simulink model "modelExperiment_QuanserAero_Hardware_AdaptiveV5"  (R2021a)
settings: Solver=ode1  StartTime=0.0  StopTime=T  FixedStep=DAQ_time  RelTol=1e-3  EnableMultiTasking=on
PreLoadFcn:
  | quanser_aero_lqr
values from neighbouring files (symbols this model uses):
  A_cmd = [Ap_cmd, Ay_cmd]    [runExperiment_QuanserAero_Hardware_AdaptiveV4_1DOF_pitch.m]    (also in runExperiment_QuanserAero_Hardware_AdaptiveV4_1DOF_yaw.m; runSim_QuanserAero_AdaptiveV3.m; run_QuanserAero_AdaptiveV3_SN.m)
  a_cmd_coeff = [ap_cmd_coeff,ay_cmd_coeff]    [runExperiment_QuanserAero_Hardware_AdaptiveV4_1DOF_pitch.m]    (also in runExperiment_QuanserAero_Hardware_AdaptiveV4_1DOF_yaw.m; runSim_QuanserAero_AdaptiveV3.m; run_QuanserAero_AdaptiveV3_SN.m)
  cmd_select = [1,0]    [runExperiment_QuanserAero_Hardware_AdaptiveV4_1DOF_pitch.m]    (also in runExperiment_QuanserAero_Hardware_AdaptiveV4_1DOF_yaw.m = [1,1]; runSim_QuanserAero_AdaptiveV3.m = [0,2]; run_QuanserAero_AdaptiveV3_SN.m = [0,2])
  control_gains = [lambda_p lambda_y ... (first row only)    [runExperiment_QuanserAero_Hardware_AdaptiveV4_1DOF_pitch.m]    (also in runExperiment_QuanserAero_Hardware_AdaptiveV4_1DOF_yaw.m; runSim_QuanserAero_AdaptiveV3.m; run_QuanserAero_AdaptiveV3_SN.m)
  gamma_p = [gamma0_p;gamma1_p;gamma2_p;gamma3_p;gamma4_p]    [runExperiment_QuanserAero_Hardware_AdaptiveV4_1DOF_pitch.m]    (also in runExperiment_QuanserAero_Hardware_AdaptiveV4_1DOF_yaw.m; runSim_QuanserAero_AdaptiveV3.m; run_QuanserAero_AdaptiveV3_SN.m)
  gamma_y = [gamma0_y;gamma1_y;gamma2_y;gamma3_y]    [runExperiment_QuanserAero_Hardware_AdaptiveV4_1DOF_pitch.m]    (also in runExperiment_QuanserAero_Hardware_AdaptiveV4_1DOF_yaw.m; runSim_QuanserAero_AdaptiveV3.m; run_QuanserAero_AdaptiveV3_SN.m)
  harmonic_cutoff_p = Tp_cmd*harmonic_cycles    (= 20)    [runExperiment_QuanserAero_Hardware_AdaptiveV4_1DOF_pitch.m]    (also in runExperiment_QuanserAero_Hardware_AdaptiveV4_1DOF_yaw.m; runSim_QuanserAero_AdaptiveV3.m; run_QuanserAero_AdaptiveV3_SN.m)
  harmonic_cutoff_y = Ty_cmd*harmonic_cycles    (= 20)    [runExperiment_QuanserAero_Hardware_AdaptiveV4_1DOF_pitch.m]    (also in runExperiment_QuanserAero_Hardware_AdaptiveV4_1DOF_yaw.m; runSim_QuanserAero_AdaptiveV3.m; run_QuanserAero_AdaptiveV3_SN.m = 40)
  paramsGuess_haaaa = [hp_hat hy_hat ... (first row only)    [runExperiment_QuanserAero_Hardware_AdaptiveV4_1DOF_pitch.m]    (also in runExperiment_QuanserAero_Hardware_AdaptiveV4_1DOF_yaw.m; runSim_QuanserAero_AdaptiveV3.m; run_QuanserAero_AdaptiveV3_SN.m)
  T_cmd = [Tp_cmd, Ty_cmd]    [runExperiment_QuanserAero_Hardware_AdaptiveV4_1DOF_pitch.m]    (also in runExperiment_QuanserAero_Hardware_AdaptiveV4_1DOF_yaw.m; runSim_QuanserAero_AdaptiveV3.m; run_QuanserAero_AdaptiveV3_SN.m)
  time_offset = 2    [runExperiment_QuanserAero_Hardware_AdaptiveV4_1DOF_pitch.m]    (also in runExperiment_QuanserAero_Hardware_AdaptiveV4_1DOF_yaw.m)
undefined symbols (not defined in the file or in its folder): HIL, qc_get_step_size
libraries: quarc_library x7
settings Model: SimulationMode=external  ExtModeTrigDuration=20000  Creator=MLevis  LastModifiedBy=Student
settings SolverCC: AlgebraicLoopSolver=TrustRegion  PositivePriorityOrder=on
settings DataIOCC: LimitDataPoints=on  SaveFormat=Array  ReturnWorkspaceOutputs=off
settings DebuggingCC: SolverPrmCheckMsg=warning  SFUnexpectedBacktrackingDiag=warning  SFNoUnconditionalDefaultTransitionDiag=warning  SFExecutionAtInitializationDiag=none  SFMachineParentedDataDiag=warning  ArithmeticOperatorsInVariantConditions=warning
settings ModelReferenceCC: PropagateSignalLabelsOutOfModel=off
settings SFSimCC: SimUseLocalCustomCode=off  CustomCodeUndefinedFunction=UseInterfaceOnly
settings RTWCC: Description=QUARC Win64 Target Using Toolchain  SystemTargetFile=quarc_win64.tlc  TemplateMakefile=quarc_default_tmf  RTWUseLocalCustomCode=off  Toolchain=QUARC win64 | nmake (64-bit Windows)  BuildConfiguration=Faster Runs
settings CodeAppCC: StateflowObjectComments=on
settings STFCustomTargetCC: ConcurrentExecutionCompliant=on  SystemTargetFile=quarc_win64.tlc
settings GRTTargetCC: TargetLangStandard=C89/C90 (ANSI)  ParMdlRefBuildCompliant=off  CompOptLevelCompliant=off  CombineOutputUpdateFcns=off  MatFileLogging=off  CPPClassGenCompliant=off  GRTInterface=on  ExtMode=on  ExtModeMexFile=quarc_comm
settings ConfigComp: CovMetricSettings=dw  CovSaveCumulativeToWorkspaceVar=on  CovSaveSingleToWorkspaceVar=on  CovExternalEMLEnable=off  CovSFcnEnable=off

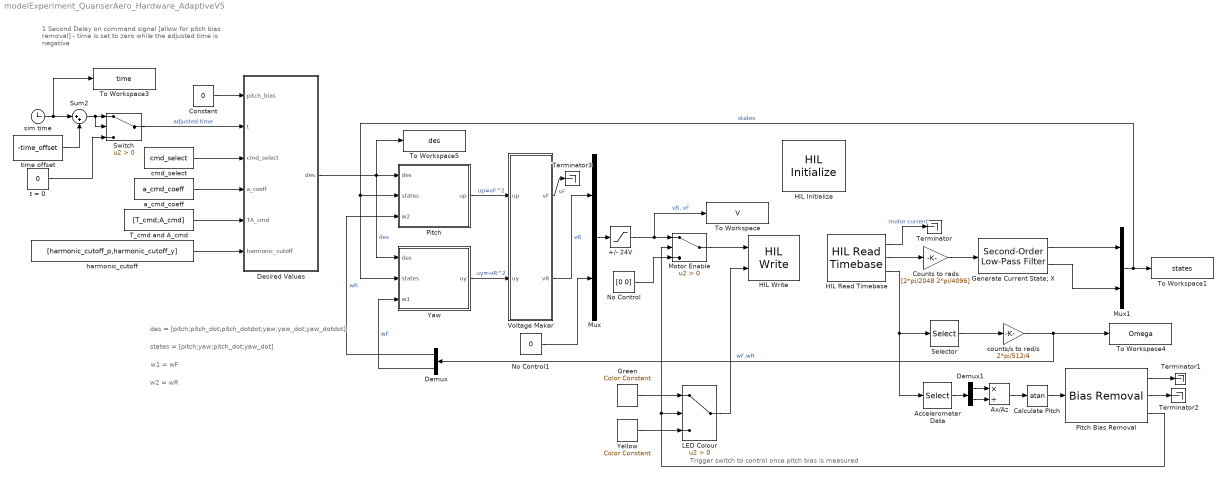
== system modelExperiment_QuanserAero_Hardware_AdaptiveV5 ==
  note: des = [pitch;pitch_dot;pitch_dotdot;yaw;yaw_dot;yaw_dotdot]
  note: w2 = wR
  note: w1 = wF
  note: 1 Second Delay on command signal
      | [allow for pitch bias removal]
      | - time is set to zero while the adjusted time is negative
  note: Trigger switch to control once pitch bias is measured
  note: states = [pitch;yaw;pitch_dot;yaw_dot]
  +/- 24V : Saturate  UpperLimit=24  LowerLimit=-24
  Accelerometer Data : Selector  InputPortWidth=4  IndexOptions=Index vector (dialog)  Indices=[1 2]  OutputSizes=1
  Ax/Az : Product  Inputs=*/
  Calculate Pitch : Trigonometry  Operator=atan
  Constant : Constant  Value=0
  Counts to rads : Gain  Gain=[2*pi/2048 2*pi/4096]
  Demux : Demux  Outputs=2
  Demux1 : Demux  Outputs=2
  Desired Values : MATLAB Function  TreatAsAtomicUnit=on
  Generate Current State; X : quarc_library/Continuous/Second-Order Low-Pass Filter  params_source=Internal (dialog parameters)  input_width=50  input_zeta=0.8  input_init=0
  Green : quarc_library/Sources/Signals/Color Constant  color=[0 1 0]
      settings: SourceProductName=QUARC Targets
  HIL Initialize : quarc_library/Data Acquisition/Generic/Configuration/HIL Initialize  Priority=-99  object_name=HIL-1  board_type=quanser_aero_usb  board_number=0  board_options=""  exclusive=off  active=off  hardware_clocks=[0]  clock_modes=[]  initial_clock_frequencies=[]  set_clock_params_at_start=off  set_clock_params_at_switch_in=off  set_clock_frequencies_at_start=off  set_clock_frequencies_at_switch_in=off  analog_input_channels=[0:1]  analog_input_configurations=[]  analog_input_maximums=3  analog_input_minimums=-3  set_analog_input_params_at_start=off  set_analog_input_params_at_switch_in=off  analog_output_channels=[0:1]  analog_output_maximums=24  analog_output_minimums=-24  initial_analog_outputs=[0]  final_analog_outputs=[0]  watchdog_analog_outputs=[0]  set_analog_output_params_at_start=off  set_analog_output_params_at_switch_in=off  set_analog_outputs_at_start=on  set_analog_outputs_at_switch_in=off  set_analog_outputs_at_terminate=on  set_analog_outputs_at_switch_out=off  set_analog_outputs_on_watchdog=on  digital_input_channels=[]  digital_output_channels=[0:1]  digital_output_configuration=[]  initial_digital_outputs=[1]  final_digital_outputs=[0]  watchdog_digital_outputs=[0]  set_digital_output_params_at_start=off  set_digital_output_params_at_switch_in=off  set_digital_outputs_at_start=on  set_digital_outputs_at_switch_in=off  set_digital_outputs_at_terminate=on  set_digital_outputs_at_switch_out=off  set_digital_outputs_on_watchdog=on  encoder_channels=[0:3]  quadrature=[4]  encoder_filter_frequency=[]  initial_encoder_counts=[0]  set_encoder_params_at_start=off  set_encoder_params_at_switch_in=off  set_encoder_counts_at_start=on  set_encoder_counts_at_switch_in=off  pwm_channels=[]  pwm_modes=[]  pwm_frequency=[]  pwm_configuration=[]  pwm_alignment=[]  pwm_polarity=[]  pwm_leading_deadband=[]  pwm_trailing_deadband=[]  initial_pwm_outputs=[]  final_pwm_outputs=[]  watchdog_pwm_outputs=[]  set_pwm_params_at_start=off  set_pwm_params_at_switch_in=off  set_pwm_outputs_at_start=off  set_pwm_outputs_at_switch_in=off  set_pwm_outputs_at_terminate=off  set_pwm_outputs_at_switch_out=off  set_pwm_outputs_on_watchdog=off  other_output_channels=[11000:11002]  initial_other_outputs=[0 1 0]  final_other_outputs=[1 0 0]  watchdog_other_outputs=[0 0 1]  set_other_outputs_at_start=on  set_other_outputs_at_switch_in=off  set_other_outputs_at_terminate=on  set_other_outputs_at_switch_out=off  set_other_outputs_on_watchdog=on
  HIL Read Timebase : quarc_library/Data Acquisition/Generic/Timebases/HIL Read Timebase  object_name=HIL-1  clock=0  analog_channels=[0:1]  encoder_channels=[2:3]  digital_channels=[]  other_channels=[4000 4002 14000 14001]  active=on  vector_output=on  data_type_mode=Inherit via back propagation  encoder_data_type=double  digital_data_type=boolean  overflow_mode=Error on overflow  samples_in_buffer=max(ceil(1/qc_get_step_size), 1)
  HIL Write : quarc_library/Data Acquisition/Generic/Immediate I//O/HIL Write  object_name=HIL-1  analog_channels=[0:1]  pwm_channels=[]  digital_channels=[]  other_channels=[11000:11002]  sample_time=-1  active=off  vector_input=on
  LED Colour : Switch  Criteria=u2 > Threshold
  Motor Enable : Switch  Criteria=u2 > Threshold
  Mux : Mux  Inputs=2
  Mux1 : Mux  Inputs=2
  No Control : Constant  Value=[0 0]
  No Control1 : Constant  Value=0
  Pitch : Subsystem
  Pitch Bias Removal : quarc_library/Discrete/Bias Removal  start_time=0  end_time=1  switch_id=0  sample_time=qc_get_step_size
      settings: SourceProductName=QUARC Targets
  Selector : Selector  InputPortWidth=4  IndexOptions=Index vector (dialog)  Indices=[3 4]  OutputSizes=1
  Sum2 : Sum  Inputs=|++
  Switch : Switch  Criteria=u2 > Threshold
  T_cmd and A_cmd : Constant  Value=[T_cmd;A_cmd]
  Terminator{,1..3} (4 alike) : Terminator
  To Workspace : ToWorkspace  VariableName=V  SampleTime=-1
  To Workspace1 : ToWorkspace  VariableName=states  SampleTime=-1
  To Workspace3 : ToWorkspace  VariableName=time  SampleTime=-1
  To Workspace4 : ToWorkspace  VariableName=Omega  SampleTime=-1
  To Workspace5 : ToWorkspace  VariableName=des  SampleTime=-1
  Voltage Maker : MATLAB Function  TreatAsAtomicUnit=on
  Yaw : Subsystem
  Yellow : quarc_library/Sources/Signals/Color Constant  color=[1 1 0]
      settings: SourceProductName=QUARC Targets
  a_cmd_coeff : Constant  Value=a_cmd_coeff
  cmd_select : Constant  Value=cmd_select
  counts/s to rad/s : Gain  Gain=2*pi/512/4
  harmonic_cutoff : Constant  Value=[harmonic_cutoff_p,harmonic_cutoff_y]
  sim time : Clock
  t = 0 : Constant  Value=0
  time offset : Constant  Value=-time_offset
  wires:
  HIL Read Timebase/2 -> Counts to rads/1
  Pitch Bias Removal/3 -> Motor Enable/2, LED Colour/2
  LED Colour/1 -> HIL Write/2
  No Control/1 -> Motor Enable/3
  Green/1 -> LED Colour/1
  Yellow/1 -> LED Colour/3
  HIL Read Timebase/3 -> Selector/1, Accelerometer Data/1
  Demux1/1 -> Ax/Az/1
  Demux1/2 -> Ax/Az/2
  Ax/Az/1 -> Calculate Pitch/1
  Calculate Pitch/1 -> Pitch Bias Removal/1
  Pitch Bias Removal/1 -> Terminator1/1
  HIL Read Timebase/1 -> Terminator/1  "motor current"
  Accelerometer Data/1 -> Demux1/1
  time offset/1 -> Sum2/2
  sim time/1 -> To Workspace3/1, Sum2/1
  Sum2/1 -> Switch/2, Switch/1
  t = 0/1 -> Switch/3
  Switch/1 -> Desired Values/2(t)  "adjusted time"
  Mux/1 -> +/- 24V/1
  Voltage Maker/1(vF) -> Terminator3/1  "vF"
  Voltage Maker/2(vR) -> Mux/1  "vR"
  Yaw/1(uy) -> Voltage Maker/2(uy)  "uy=-vR^2"
  Pitch/1(up) -> Voltage Maker/1(up)  "up=vF^2"
  T_cmd and A_cmd/1 -> Desired Values/5(TA_cmd)
  harmonic_cutoff/1 -> Desired Values/6(harmonic_cutoff)
  cmd_select/1 -> Desired Values/3(cmd_select)
  a_cmd_coeff/1 -> Desired Values/4(a_coeff)
  Desired Values/1(des) -> To Workspace5/1, Pitch/1(des), Yaw/1(des)  "des"
  Selector/1 -> counts/s to rad/s/1
  counts/s to rad/s/1 -> Demux/1, To Workspace4/1  "wF,wR"
  Counts to rads/1 -> Generate Current State; X/1
  Mux1/1 -> To Workspace1/1, Pitch/2(states), Yaw/2(states)  "states"
  Pitch Bias Removal/2 -> Terminator2/1
  Constant/1 -> Desired Values/1(pitch_bias)
  +/- 24V/1 -> To Workspace/1, Motor Enable/1  "vR, vF"
  Demux/2 -> Yaw/3(w1)  "wF"
  Demux/1 -> Pitch/3(w2)  "wR"
  Motor Enable/1 -> HIL Write/1
  Generate Current State; X/2 -> Mux1/2
  Generate Current State; X/1 -> Mux1/1
  No Control1/1 -> Mux/2

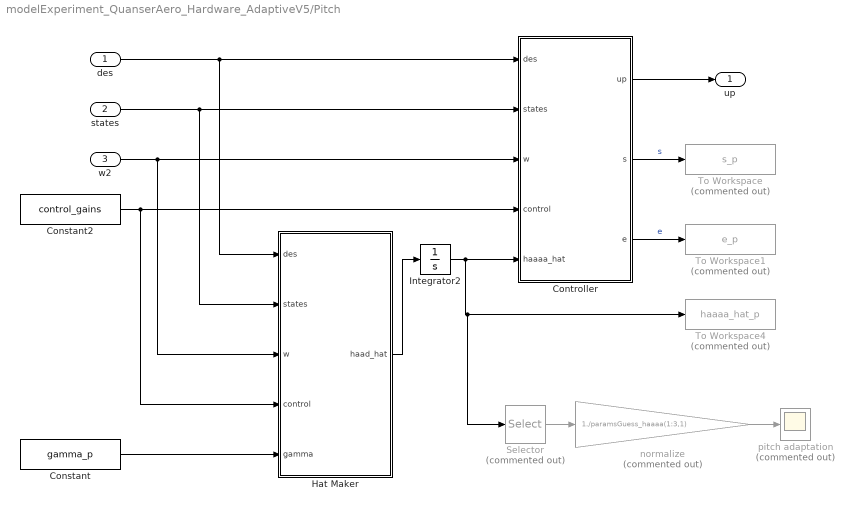
== system modelExperiment_QuanserAero_Hardware_AdaptiveV5/Pitch ==
  des : Inport
  states : Inport  Port=2
  w2 : Inport  Port=3
  Constant : Constant  Value=gamma_p
  Constant2 : Constant  Value=control_gains
  Controller : MATLAB Function  TreatAsAtomicUnit=on
  Hat Maker : MATLAB Function  TreatAsAtomicUnit=on
  Integrator2 : Integrator  InitialCondition=paramsGuess_haaaa(:,1)
  Selector : Selector  Commented=on  InputPortWidth=5  IndexOptions=Index vector (dialog)  Indices=[1 2 3]  OutputSizes=1
  To Workspace : ToWorkspace  Commented=on  VariableName=s_p  SampleTime=-1
  To Workspace1 : ToWorkspace  Commented=on  VariableName=e_p  SampleTime=-1
  To Workspace4 : ToWorkspace  Commented=on  VariableName=haaaa_hat_p  SampleTime=-1
  normalize : Gain  Commented=on  Gain=1./paramsGuess_haaaa(1:3,1)
  pitch adaptation : Scope  Commented=on
  up : Outport
  wires:
  Integrator2/1 -> Selector/1, To Workspace4/1, Controller/5(haaaa_hat)
  Hat Maker/1(haad_hat) -> Integrator2/1
  Controller/1(up) -> up/1
  states/1 -> Hat Maker/2(states), Controller/2(states)
  Controller/2(s) -> To Workspace/1  "s"
  des/1 -> Hat Maker/1(des), Controller/1(des)
  w2/1 -> Hat Maker/3(w), Controller/3(w)
  Constant2/1 -> Hat Maker/4(control), Controller/4(control)
  Constant/1 -> Hat Maker/5(gamma)
  Controller/3(e) -> To Workspace1/1  "e"
  normalize/1 -> pitch adaptation/1
  Selector/1 -> normalize/1

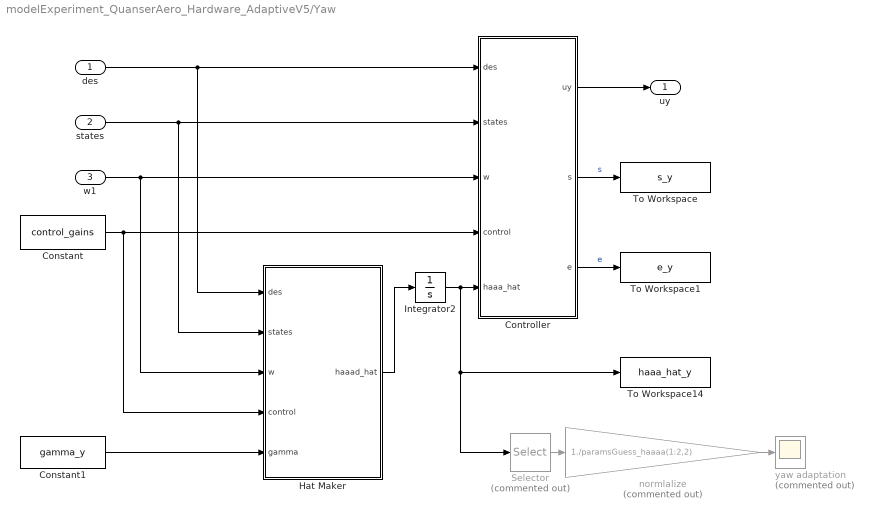
== system modelExperiment_QuanserAero_Hardware_AdaptiveV5/Yaw ==
  des : Inport
  states : Inport  Port=2
  w1 : Inport  Port=3
  Constant : Constant  Value=control_gains
  Constant1 : Constant  Value=gamma_y
  Controller : MATLAB Function  TreatAsAtomicUnit=on
  Hat Maker : MATLAB Function  TreatAsAtomicUnit=on
  Integrator2 : Integrator  InitialCondition=paramsGuess_haaaa(1:4,2)
  Selector : Selector  Commented=on  InputPortWidth=4  IndexOptions=Index vector (dialog)  Indices=[1 2]  OutputSizes=1
  To Workspace : ToWorkspace  VariableName=s_y  SampleTime=-1
  To Workspace1 : ToWorkspace  VariableName=e_y  SampleTime=-1
  To Workspace14 : ToWorkspace  VariableName=haaa_hat_y  SampleTime=-1
  normlalize : Gain  Commented=on  Gain=1./paramsGuess_haaaa(1:2,2)
  yaw adaptation : Scope  Commented=on
  uy : Outport
  wires:
  des/1 -> Controller/1(des), Hat Maker/1(des)
  Hat Maker/1(haaad_hat) -> Integrator2/1
  Controller/1(uy) -> uy/1
  Controller/2(s) -> To Workspace/1  "s"
  states/1 -> Controller/2(states), Hat Maker/2(states)
  w1/1 -> Hat Maker/3(w), Controller/3(w)
  Controller/3(e) -> To Workspace1/1  "e"
  Constant/1 -> Hat Maker/4(control), Controller/4(control)
  Constant1/1 -> Hat Maker/5(gamma)
  Integrator2/1 -> To Workspace14/1, Selector/1, Controller/5(haaa_hat)
  normlalize/1 -> yaw adaptation/1
  Selector/1 -> normlalize/1

== matlab function modelExperiment_QuanserAero_Hardware_AdaptiveV5/Voltage Maker ==
  data: up input; vF output; uy input; vR output
function [vF,vR] = fcn(up,uy)
% convert controller ouput to plant input (voltage)
vF = sqrt(abs(up))*sign(up);
vR = -sqrt(abs(uy))*sign(uy);

== matlab function modelExperiment_QuanserAero_Hardware_AdaptiveV5/Desired Values ==
  data: pitch_bias input; t input; des output; cmd_select input; a_coeff input; TA_cmd input; harmonic_cutoff input
function des = fcn(pitch_bias, t,cmd_select,a_coeff,TA_cmd,harmonic_cutoff)
%% initialize outputs
des = zeros(6,1);

%% input parameters
ap_coeff = a_coeff(:,1); % polynomial coefficients for smooth step function
ay_coeff = a_coeff(:,2); % polynomial coefficients for smooth step function
Tp = TA_cmd(1,1); % pitch command period
Ty = TA_cmd(1,2); % yaw command period
PitchMag = TA_cmd(2,1); % pitch command amplitude
YawMag = TA_cmd(2,2); % yaw command amplitude
step_cos = cmd_select(1); % smooth step input or harmonic oscilator input selection
py_on_off = cmd_select(2); % pitch and yaw on or off selection
harmonic_cutoff_p = harmonic_cutoff(1); % time to command zero position, velocity, acceleration
harmonic_cutoff_y = harmonic_cutoff(2); % time to command zero position, velocity, acceleration

%% functions
if py_on_off == 0
    if step_cos == 0
        if t <= Tp
            pitch_des = ap_coeff(1)*t^4 + ap_coeff(2)*t^5 + ap_coeff(3)*t^6 + ap_coeff(4)*t^7;
            pitchd_des = 4*ap_coeff(1)*t^3 + 5*ap_coeff(2)*t^4 + 6*ap_coeff(3)*t^5 + 7*ap_coeff(4)*t^6;
            pitchdd_des = 12*ap_coeff(1)*t^2 + 20*ap_coeff(2)*t^3 + 30*ap_coeff(3)*t^4 + 42*ap_coeff(4)*t^5;
        else
            pitch_des = PitchMag;
            pitchd_des = 0;
            pitchdd_des = 0;
        end
        yaw_des = 0;
        yawd_des = 0;
        yawdd_des = 0;
    elseif step_cos == 1 && t<harmonic_cutoff_p
        pitch_des = (PitchMag/2)*(1-cos(2*pi*t/Tp));
        pitchd_des = (2*pi/Tp)*(PitchMag/2)*sin(2*pi*t/Tp);
        pitchdd_des = (2*pi/Tp)^2*(PitchMag/2)*cos(2*pi*t/Tp);
        yaw_des = 0;
        yawd_des = 0;
        yawdd_des = 0;
    elseif step_cos == 1 && t>=harmonic_cutoff_p
        pitch_des = 0;
        pitchd_des = 0;
        pitchdd_des = 0;
        yaw_des = 0;
        yawd_des = 0;
        yawdd_des = 0;
    else
        error("Not A Valid cmd_select")
    end
elseif py_on_off == 1
    if step_cos == 0
        pitch_des =0;
        pitchd_des = 0;
        pitchdd_des = 0;
        if t <= Ty
            yaw_des = ay_coeff(1)*t^4 + ay_coeff(2)*t^5 + ay_coeff(3)*t^6 + ay_coeff(4)*t^7;
            yawd_des = 4*ay_coeff(1)*t^3 + 5*ay_coeff(2)*t^4 + 6*ay_coeff(3)*t^5 + 7*ay_coeff(4)*t^6;
            yawdd_des = 12*ay_coeff(1)*t^2 + 20*ay_coeff(2)*t^3 + 30*ay_coeff(3)*t^4 + 42*ay_coeff(4)*t^5;
        else
            yaw_des = YawMag;
            yawd_des = 0;
            yawdd_des = 0;
        end
    elseif step_cos == 1 && t<harmonic_cutoff_y
        pitch_des =0;
        pitchd_des = 0;
        pitchdd_des = 0;
        yaw_des = (YawMag/2)*(1-cos(2*pi*t/Ty));
        yawd_des = (2*pi/Ty)*(YawMag/2)*sin(2*pi*t/Ty);
        yawdd_des = (2*pi/Ty)^2*(YawMag/2)*cos(2*pi*t/Ty);
    elseif step_cos == 1 && t>=harmonic_cutoff_y
        pitch_des =0;
        pitchd_des = 0;
        pitchdd_des = 0;
        yaw_des = 0;
        yawd_des = 0;
        yawdd_des = 0;
    else
        error("Not A Valid cmd_select")
    end
elseif py_on_off == 2
    if step_cos == 0
        if t <= Tp
            pitch_des = ap_coeff(1)*t^4 + ap_coeff(2)*t^5 + ap_coeff(3)*t^6 + ap_coeff(4)*t^7;
            pitchd_des = 4*ap_coeff(1)*t^3 + 5*ap_coeff(2)*t^4 + 6*ap_coeff(3)*t^5 + 7*ap_coeff(4)*t^6;
            pitchdd_des = 12*ap_coeff(1)*t^2 + 20*ap_coeff(2)*t^3 + 30*ap_coeff(3)*t^4 + 42*ap_coeff(4)*t^5;
        else
            pitch_des = PitchMag;
            pitchd_des = 0;
            pitchdd_des = 0;
        end
        if t <= Ty
            yaw_des = ay_coeff(1)*t^4 + ay_coeff(2)*t^5 + ay_coeff(3)*t^6 + ay_coeff(4)*t^7;
            yawd_des = 4*ay_coeff(1)*t^3 + 5*ay_coeff(2)*t^4 + 6*ay_coeff(3)*t^5 + 7*ay_coeff(4)*t^6;
            yawdd_des = 12*ay_coeff(1)*t^2 + 20*ay_coeff(2)*t^3 + 30*ay_coeff(3)*t^4 + 42*ay_coeff(4)*t^5;
        else
            yaw_des = YawMag;
            yawd_des = 0;
            yawdd_des = 0;
        end
    elseif  step_cos == 1
        if t<harmonic_cutoff_p
            pitch_des = (PitchMag/2)*(1-cos(2*pi*t/Tp));
            pitchd_des = (2*pi/Tp)*(PitchMag/2)*sin(2*pi*t/Tp);
            pitchdd_des = (2*pi/Tp)^2*(PitchMag/2)*cos(2*pi*t/Tp);
        else
            pitch_des = 0;
            pitchd_des = 0;
            pitchdd_des = 0;
        end
        if t<harmonic_cutoff_p
            yaw_des = (YawMag/2)*(1-cos(2*pi*t/Ty));
            yawd_des = (2*pi/Ty)*(YawMag/2)*sin(2*pi*t/Ty);
            yawdd_des = (2*pi/Ty)^2*(YawMag/2)*cos(2*pi*t/Ty);
        else
            yaw_des = 0;
            yawd_des = 0;
            yawdd_des = 0;
        end
    else
        error("Not A Valid cmd_select")
    end
else
    error("Not A Valid cmd_select")
end

des = [pitch_des-pitch_bias;
       pitchd_des;
       pitchdd_des
       yaw_des;
       yawd_des;
       yawdd_des];

== matlab function modelExperiment_QuanserAero_Hardware_AdaptiveV5/Pitch/Controller ==
  data: des input; states input; w input; control input; up output; haaaa_hat input; s output; e output
function [up,s,e]= fcn(des,states,w,control,haaaa_hat)
%% initialize outputs
up = zeros(1,1);
s = zeros(1,1);
e = zeros(1,1);

%% separate input vectors
% desired variables
r_pitch_des = des(1,1);
rd_pitch_des = des(2,1);
rdd_pitch_des = des(3,1);
% state variables
r_pitch = states(1,1);
% state derivative variables
rd_pitch = states(3,1);
% motor angular speed
r_omega_r = w;
% controller gains
lambda = control(1,1);
D = control(2,1);
eta = control(3,1);
phi_para = control(4,1);
% estimated parameters
h_hat = haaaa_hat(1,1);
a1_hat = haaaa_hat(2,1);
a2_hat = haaaa_hat(3,1);
a3_hat = haaaa_hat(4,1);
a4_hat = haaaa_hat(5,1);

%% functions
e = r_pitch-r_pitch_des;
ed = rd_pitch-rd_pitch_des;
rdd_pitch_ref = rdd_pitch_des - lambda*ed; %+ 2*lambda*ed + lambda^2*e;
s = ed + lambda*e;

if abs(s)>phi_para
    sat = sign(s);
else
    sat = s/phi_para;
end

f1 = rd_pitch;
f2 = sin(r_pitch);
f3 = r_omega_r;
f4 = sign(r_omega_r)*r_omega_r^2;

%% outputs
up = -h_hat*(D+eta)*sat + h_hat*rdd_pitch_ref + a1_hat*f1 + a2_hat*f2 ...
                                              + a3_hat*f3 + a4_hat*f4;

== matlab function modelExperiment_QuanserAero_Hardware_AdaptiveV5/Pitch/Hat Maker ==
  data: des input; states input; haad_hat output; w input; control input; gamma input
function haad_hat = fcn(des,states,w,control,gamma)
%% initialize outputs
haad_hat = zeros(5,1);

%% separate input vectors
% desired variables
r_pitch_des = des(1,1);
rd_pitch_des = des(2,1);
rdd_pitch_des = des(3,1);
% state variables
r_pitch = states(1,1);
% state derivative variables
rd_pitch = states(3,1);
% motor angular speed
r_omega_r = w;
% controller gains
lambda = control(1,1);
D = control(2,1);
eta = control(3,1);
phi_para = control(4,1);
gamma_0 = gamma(1,1);
gamma_1 = gamma(2,1);
gamma_2 = gamma(3,1);
gamma_3 = gamma(4,1);
gamma_4 = gamma(5,1);

%% functions
e = r_pitch-r_pitch_des;
ed = rd_pitch-rd_pitch_des;
rdd_pitch_ref = rdd_pitch_des - lambda*ed; %+ 2*lambda*ed + lambda^2*e;
s = ed + lambda*e;

if abs(s)>phi_para
    sat = sign(s);
else
    sat = s/phi_para;
end
s_delta = s - (phi_para * sat);

f1 = rd_pitch;
f2 = sin(r_pitch);
f3 = r_omega_r;
f4 = sign(r_omega_r)*r_omega_r^2;

%% outputs
hd_hat  = gamma_0^2 * s_delta * (rdd_pitch_ref + ((D + eta) * sat));
a1d_hat = -gamma_1^2 * s_delta * f1;
a2d_hat = -gamma_2^2 * s_delta * f2;
a3d_hat = -gamma_3^2 * s_delta * f3;
a4d_hat = -gamma_4^2 * s_delta * f4;
haad_hat = [hd_hat;
            a1d_hat;
            a2d_hat;
            a3d_hat;
            a4d_hat];

== matlab function modelExperiment_QuanserAero_Hardware_AdaptiveV5/Yaw/Controller ==
  data: des input; states input; w input; control input; uy output; haaa_hat input; s output; e output
function [uy,s,e]= fcn(des,states,w,control,haaa_hat)
%% initialize outputs
uy = zeros(1,1);
s = zeros(1,1);
e = zeros(1,1);

%% separate input vectors
% desired variables
yaw_des = des(4,1);
yawd_des = des(5,1);
yawdd_des = des(6,1);
% state variables
r_yaw = states(2,1);
% state derivative variables
rd_yaw = states(4,1);
% motor angular speed
r_omega_f = w;
% controller gains
lambda = control(1,2);
D = control(2,2);
eta = control(3,2);
phi_para = control(4,2);
% parameter estimations
h_hat = haaa_hat(1,1);
a1_hat = haaa_hat(2,1);
a2_hat = haaa_hat(3,1);
a3_hat = haaa_hat(4,1);

%% functions
e = r_yaw-yaw_des;
ed = rd_yaw-yawd_des;
yawdd_ref = yawdd_des - lambda*ed;
s = ed + lambda*e;

if abs(s)>phi_para
    sat = sign(s);
else
    sat = s/phi_para;
end

f1 = rd_yaw;
f2 = r_omega_f;
f3 = sign(r_omega_f)*r_omega_f^2;

%% outputs
uy = -h_hat*(D+eta)*sat + h_hat*yawdd_ref + a1_hat*f1 + a2_hat*f2 ...
                                                      + a3_hat*f3;

== matlab function modelExperiment_QuanserAero_Hardware_AdaptiveV5/Yaw/Hat Maker ==
  data: des input; states input; haaad_hat output; w input; control input; gamma input
function haaad_hat = fcn(des,states,w,control,gamma)
%% initialize outputs
haaad_hat = zeros(4,1);

%% separate input vectors
% desired variables
yaw_des = des(4,1);
yawd_des = des(5,1);
yawdd_des = des(6,1);
% state variables
r_yaw = states(2,1);
% state derivative variables
rd_yaw = states(4,1);
% motor angular velocity
r_omega_f = w;
% controller gains
lambda = control(1,2);
D = control(2,2);
eta = control(3,2);
phi_para = control(4,2);
gamma_0 = gamma(1,1);
gamma_1 = gamma(2,1);
gamma_2 = gamma(3,1);
gamma_3 = gamma(4,1);

%% functions
e = r_yaw-yaw_des;
ed = rd_yaw-yawd_des;
yawdd_ref = yawdd_des - lambda*ed; %2*lambda*ed + lambda^2*e;
s = ed + lambda*e;

%saturation function
% if s>phi_para
%   sat = 1;
% elseif (s>=-phi_para)&&(s<=phi_para)
%   sat = s/phi_para;
% else
%   sat = -1;
% end
if abs(s)>phi_para
    sat = sign(s);
else
    sat = s/phi_para;
end
s_delta = s - (phi_para * sat);

f1 = rd_yaw;
f2 = r_omega_f;
f3 = sign(r_omega_f)*r_omega_f^2;

%% outputs
hd_hat  = gamma_0^2 * s_delta * (yawdd_ref + ((D + eta) * sat));
a1d_hat = -gamma_1^2 * s_delta * f1;
a2d_hat = -gamma_2^2 * s_delta * f2;
a3d_hat = -gamma_3^2 * s_delta * f3;
haaad_hat = [hd_hat;a1d_hat;a2d_hat;a3d_hat];
